simulink model "te_plant"  (R2013b)
settings: Solver=ode5  SolverMode=SingleTasking  StartTime=0.0  StopTime=15  FixedStep=Ts_base  MaxStep=Ts_base  MinStep=1e-6  RelTol=1e-6
InitFcn:
  | global model_type
  | model_type = -1  % plant and controller
  | 
  | init_model
StopFcn:
  | %TEplot
values from neighbouring files (symbols this model uses):
  Ts_save = Ts_base    (= 0.000277777777778)    [init_model.m]
libraries: TEsim_utils x1
settings Model: Creator=rnc4  LastModifiedBy=rnc4
settings DataIOCC: LimitDataPoints=off  LoadInitialState=on  SaveFinalState=on  SaveFormat=Structure  SignalLoggingSaveFormat=ModelDataLogs  SaveOutput=off  SaveTime=off  SignalLoggingName=sigsOut
settings OptimizationCC: InitFltsAndDblsToZero=on
settings DebuggingCC: SaveWithParameterizedLinksMsg=none  SignalResolutionControl=TryResolveAllWithWarning  SolverPrmCheckMsg=none  MultiTaskDSMMsg=warning  MultiTaskCondExecSysMsg=none  FcnCallInpInsideContextMsg=UseLocalSettings
settings HardwareCC: TargetUnknown=on
settings RTWCC: IncludeERTFirstTime=on
settings GRTTargetCC: TargetFcnLib=ansi_tfl_tmw.mat  CodeReplacementLibrary=None  CombineOutputUpdateFcns=off  CPPClassGenCompliant=on  GRTInterface=on

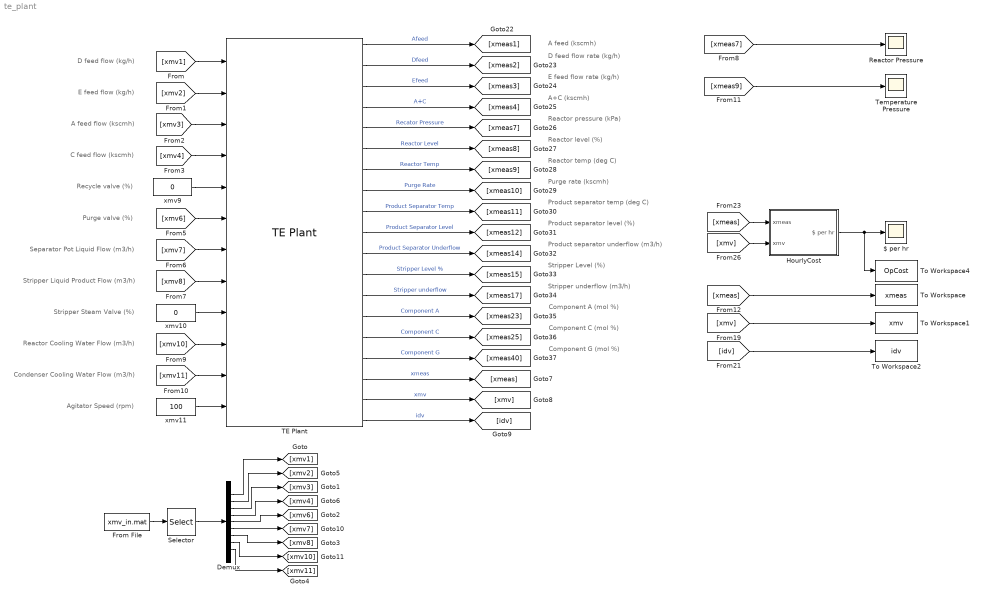
== system te_plant ==
  note: Agitator Speed (rpm)
  note: Condenser Cooling Water Flow (m3/h)
  note: Reactor Cooling Water Flow (m3/h)
  note: Stripper Steam Valve (%)
  note: Stripper Liquid Product Flow (m3/h)
  note: Separator Pot Liquid Flow (m3/h)
  note: Purge valve (%)
  note: Recycle valve (%)
  note: C feed flow (kscmh)
  note: A feed flow (kscmh)
  note: E feed flow (kg/h)
  note: D feed flow (kg/h)
  note: Component G (mol %)
  note: Component C (mol %)
  note: Component A (mol %)
  note: Stripper underflow (m3/h)
  note: Stripper Level (%)
  note: Product separator underflow (m3/h)
  note: Product separator level (%)
  note: Product separator temp (deg C)
  note: Purge rate (kscmh)
  note: Reactor temp (deg C)
  note: Reactor level (%)
  note: Reactor pressure (kPa)
  note: A+C (kscmh)
  note: E feed flow rate (kg/h)
  note: D feed flow rate (kg/h)
  note: A feed (kscmh)
  $ per hr : Scope
      settings: YMin=75  YMax=400  SaveName=OpCost  SampleInput=on  SampleTime=Ts_save
  Demux : Demux  Outputs=9
  From File : FromFile  FileName=xmv_in.mat
  HourlyCost : Subsystem
  Reactor Pressure : Scope
      settings: TimeRange=15  YMin=2795  YMax=2803.5  SampleInput=on  SampleTime=Ts_save
  Selector : Selector  InputPortWidth=41  IndexOptions=Index vector (dialog)  Indices=[1:4, 6:8, 10:11]  OutputSizes=1
  TE Plant : TEsim_utils/TEsim/TE Plant  SystemSampleTime=-1
  Temperature Pressure : Scope
      settings: TimeRange=15  YMin=122.85  YMax=122.95  SampleInput=on  SampleTime=Ts_save
  To Workspace : ToWorkspace  VariableName=xmeas  SampleTime=Ts_save
  To Workspace1 : ToWorkspace  VariableName=xmv  SampleTime=Ts_save
  To Workspace2 : ToWorkspace  VariableName=idv  SampleTime=Ts_save
  To Workspace4 : ToWorkspace  VariableName=OpCost  SampleTime=Ts_save
  xmv10 : Constant  Value=0
  xmv11 : Constant  Value=100
  xmv9 : Constant  Value=0
  wires:
  HourlyCost/1($ per hr) -> To Workspace4/1, $ per hr/1
  TE Plant/7 -> [xmeas9]  "Reactor Temp"
  TE Plant/5 -> [xmeas7]  "Recator Pressure"
  TE Plant/18 -> [xmv]  "xmv"
  TE Plant/17 -> [xmeas]  "xmeas"
  [xmv1] -> TE Plant/1
  [xmv2] -> TE Plant/2
  [xmv3] -> TE Plant/3
  [xmv4] -> TE Plant/4
  xmv9/1 -> TE Plant/5
  [xmv6] -> TE Plant/6
  [xmv7] -> TE Plant/7
  [xmv8] -> TE Plant/8
  xmv10/1 -> TE Plant/9
  [xmv10] -> TE Plant/10
  [xmv11] -> TE Plant/11
  xmv11/1 -> TE Plant/12
  TE Plant/1 -> [xmeas1]  "Afeed"
  TE Plant/2 -> [xmeas2]  "Dfeed"
  TE Plant/3 -> [xmeas3]  "Efeed"
  TE Plant/4 -> [xmeas4]  "A+C"
  TE Plant/6 -> [xmeas8]  "Reactor Level"
  TE Plant/8 -> [xmeas10]  "Purge Rate"
  TE Plant/9 -> [xmeas11]  "Product Separator Temp"
  TE Plant/10 -> [xmeas12]  "Product Separator Level"
  TE Plant/11 -> [xmeas14]  "Product Separator Underflow"
  TE Plant/12 -> [xmeas15]  "Stripper Level %"
  TE Plant/13 -> [xmeas17]  "Stripper underflow"
  TE Plant/14 -> [xmeas23]  "Component A"
  TE Plant/15 -> [xmeas25]  "Component C"
  TE Plant/16 -> [xmeas40]  "Component G"
  TE Plant/19 -> [idv]  "idv"
  [xmeas7] -> Reactor Pressure/1
  [xmeas9] -> Temperature Pressure/1
  [xmeas] -> To Workspace/1
  [xmv] -> To Workspace1/1
  [idv] -> To Workspace2/1
  [xmeas] -> HourlyCost/1(xmeas)
  [xmv] -> HourlyCost/2(xmv)
  From File/1 -> Selector/1
  Demux/1 -> [xmv1]
  Demux/2 -> [xmv2]
  Demux/3 -> [xmv3]
  Demux/4 -> [xmv4]
  Demux/5 -> [xmv6]
  Demux/6 -> [xmv7]
  Demux/7 -> [xmv8]
  Demux/8 -> [xmv10]
  Demux/9 -> [xmv11]
  Selector/1 -> Demux/1

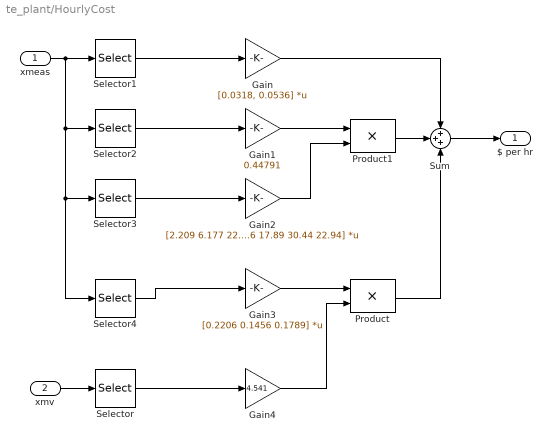
== system te_plant/HourlyCost ==
  xmeas : Inport  PortDimensions=41
  xmv : Inport  Port=2  PortDimensions=12
  Gain : Gain  Gain=[0.0318, 0.0536]  Multiplication=Matrix(K*u)  SaturateOnIntegerOverflow=on  OutDataTypeStr=Inherit: Same as input  ParamDataTypeStr=Inherit: Same as input
      settings: AttributesFormatString=%<Gain>
  Gain1 : Gain  Gain=0.44791  SaturateOnIntegerOverflow=on  OutDataTypeStr=Inherit: Same as input  ParamDataTypeStr=Inherit: Same as input
      settings: AttributesFormatString=%<Gain>
  Gain2 : Gain  Gain=[2.209 6.177 22.06 14.56 17.89 30.44 22.94]  Multiplication=Matrix(K*u)  SaturateOnIntegerOverflow=on  OutDataTypeStr=Inherit: Same as input  ParamDataTypeStr=Inherit: Same as input
      settings: AttributesFormatString=%<Gain>
  Gain3 : Gain  Gain=[0.2206 0.1456 0.1789]  Multiplication=Matrix(K*u)  SaturateOnIntegerOverflow=on  OutDataTypeStr=Inherit: Same as input  ParamDataTypeStr=Inherit: Same as input
      settings: AttributesFormatString=%<Gain>
  Gain4 : Gain  Gain=4.541  SaturateOnIntegerOverflow=on  OutDataTypeStr=Inherit: Same as input  ParamDataTypeStr=Inherit: Same as input
      settings: AttributesFormatString=%<Gain>
  Product : Product  SaturateOnIntegerOverflow=on  OutDataTypeStr=Inherit: Same as first input
  Product1 : Product  SaturateOnIntegerOverflow=on  OutDataTypeStr=Inherit: Same as first input
  Selector : Selector  InputPortWidth=12  IndexOptions=Index vector (dialog)  Indices=8  OutputSizes=1
  Selector1 : Selector  InputPortWidth=41  IndexOptions=Index vector (dialog)  Indices=[19 20]  OutputSizes=1
  Selector2 : Selector  InputPortWidth=41  IndexOptions=Index vector (dialog)  Indices=[10]  OutputSizes=1
  Selector3 : Selector  InputPortWidth=41  IndexOptions=Index vector (dialog)  Indices=[29, 31:36]  OutputSizes=1
  Selector4 : Selector  InputPortWidth=41  IndexOptions=Index vector (dialog)  Indices=[37:39]  OutputSizes=1
  Sum : Sum  Inputs=+++  SaturateOnIntegerOverflow=on
  $ per hr : Outport
  wires:
  xmv/1 -> Selector/1
  xmeas/1 -> Selector1/1, Selector2/1, Selector3/1, Selector4/1
  Selector1/1 -> Gain/1
  Selector2/1 -> Gain1/1
  Selector3/1 -> Gain2/1
  Selector4/1 -> Gain3/1
  Selector/1 -> Gain4/1
  Gain3/1 -> Product/1
  Gain4/1 -> Product/2
  Sum/1 -> $ per hr/1
  Product/1 -> Sum/3
  Gain/1 -> Sum/1
  Product1/1 -> Sum/2
  Gain1/1 -> Product1/1
  Gain2/1 -> Product1/2
